simulink model "Ejercicio8_30_03_17cont"  (R2013a)
settings: Solver=ode23tb  StartTime=0.0  StopTime=0.1  RelTol=1e-3
libraries: powerlib x34
settings Model: Creator=Miguel  LastModifiedBy=Miguel

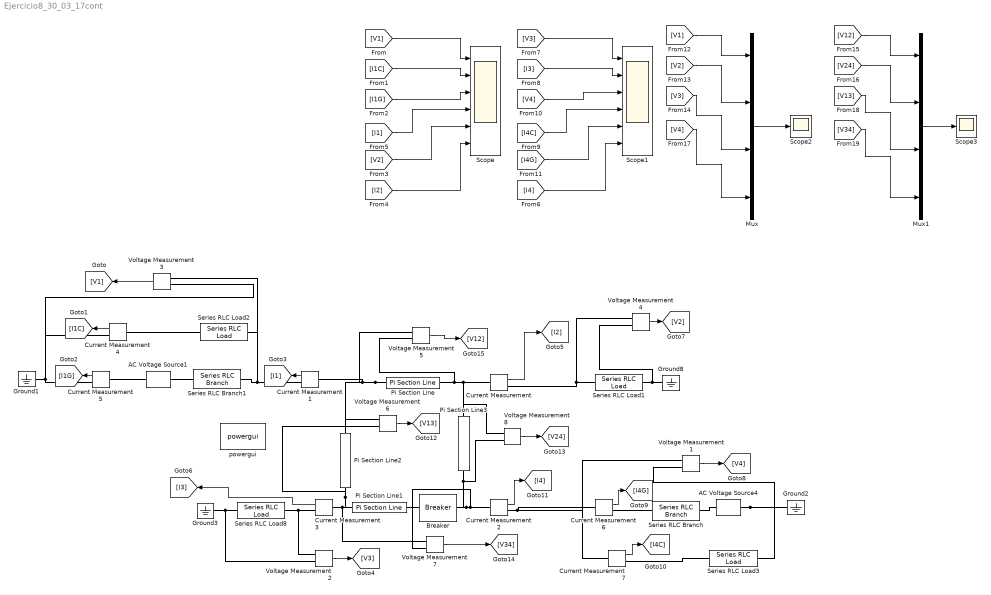
== system Ejercicio8_30_03_17cont ==
  AC Voltage Source1 : powerlib/Electrical Sources/AC Voltage Source  Amplitude=150e3*sqrt(2)  Phase=0  Frequency=60  SampleTime=0  Measurements=None
  AC Voltage Source4 : powerlib/Electrical Sources/AC Voltage Source  Amplitude=1.02*sqrt(2)*150e3  Phase=1.5231  Frequency=60  SampleTime=0  Measurements=None
  Breaker : powerlib/Elements/Breaker  BreakerResistance=0.01  InitialState=1  SnubberResistance=1e6  SnubberCapacitance=inf  SwitchingTimes=[ 1/60 ]  External=off  Measurements=None  MoreParameters=off  NoBreakLoop=off
  Current Measurement{,1..7} (8 alike) : powerlib/Measurements/Current Measurement  PhasorSimulation=off  OutputType=Complex  PSBequivalent=0
  Ground{1..3,8} (4 alike) : powerlib/Elements/Ground  LConnTagsString=a
  Mux : Mux
  Mux1 : Mux
  Pi Section Line : powerlib/Elements/Pi Section Line  LConnTagsString=__new0  RConnTagsString=__new0  Frequency=60  Resistance=0.01008*225  Inductance=0.05040/(2*pi*60)*225  Capacitance=0.05125/(pi*60*225)  Length=1  PiSections=10  Measurements=None
      settings: AttributesFormatString=\n
  Pi Section Line1 : powerlib/Elements/Pi Section Line  LConnTagsString=__new0  RConnTagsString=__new0  Frequency=60  Resistance=0.01272*225  Inductance=0.06360/(2*pi*60)*225  Capacitance=0.06375/(pi*60*225)  Length=1  PiSections=10  Measurements=All voltages and currents
      settings: AttributesFormatString=\n
  Pi Section Line2 : powerlib/Elements/Pi Section Line  LConnTagsString=__new0  RConnTagsString=__new0  Frequency=60  Resistance=0.00744*225  Inductance=0.03720/(2*pi*60)*225  Capacitance=0.03875/(pi*60*225)  Length=1  PiSections=10  Measurements=All voltages and currents
      settings: AttributesFormatString=\n
  Pi Section Line3 : powerlib/Elements/Pi Section Line  LConnTagsString=__new0  RConnTagsString=__new0  Frequency=60  Resistance=0.00744*225  Inductance=0.03720/(2*pi*60)*225  Capacitance=0.03875/(pi*60*225)  Length=1  PiSections=10  Measurements=None
      settings: AttributesFormatString=\n
  Scope : Scope  NumInputPorts=6
      settings: ShowLegends=on  YMin=-5~-5~-5~-5~-5~-5  YMax=5~5~5~5~5~5
  Scope1 : Scope  NumInputPorts=6
      settings: ShowLegends=on  YMin=-5~-5~-5~-5~-5~-5  YMax=5~5~5~5~5~5
  Scope2 : Scope
      settings: ShowLegends=on  SaveName=ScopeData2
  Scope3 : Scope
      settings: ShowLegends=on  SaveName=ScopeData3
  Series RLC Branch : powerlib/Elements/Series RLC Branch  LConnTagsString=__new0  RConnTagsString=__new0  BranchType=R  Resistance=1e-9  Inductance=1e-3  SetiL0=off  InitialCurrent=0  Capacitance=1e-6  Setx0=off  InitialVoltage=0  Measurements=None
  Series RLC Branch1 : powerlib/Elements/Series RLC Branch  LConnTagsString=__new0  RConnTagsString=__new0  BranchType=R  Resistance=1e-9  Inductance=1e-3  SetiL0=off  InitialCurrent=0  Capacitance=1e-6  Setx0=off  InitialVoltage=0  Measurements=None
  Series RLC Load1 : powerlib/Elements/Series RLC Load  LConnTagsString=a  RConnTagsString=__new0  NominalVoltage=0.9824*150e3  NominalFrequency=60  ActivePower=170e6  InductivePower=105.35e6  CapacitivePower=0  Setx0=off  InitialVoltage=0  SetiL0=off  InitialCurrent=0  Measurements=None
  Series RLC Load2 : powerlib/Elements/Series RLC Load  LConnTagsString=a  RConnTagsString=__new0  NominalVoltage=150e3  NominalFrequency=60  ActivePower=50e6  InductivePower=30.99e6  CapacitivePower=0  Setx0=off  InitialVoltage=0  SetiL0=off  InitialCurrent=0  Measurements=None
  Series RLC Load3 : powerlib/Elements/Series RLC Load  LConnTagsString=a  RConnTagsString=__new0  NominalVoltage=1.02*150e3  NominalFrequency=60  ActivePower=80e6  InductivePower=49.59e6  CapacitivePower=0  Setx0=off  InitialVoltage=0  SetiL0=off  InitialCurrent=0  Measurements=None
  Series RLC Load8 : powerlib/Elements/Series RLC Load  LConnTagsString=a  RConnTagsString=__new0  NominalVoltage=0.9690*150e3  NominalFrequency=60  ActivePower=200e6  InductivePower=123.94e6  CapacitivePower=0  Setx0=off  InitialVoltage=0  SetiL0=off  InitialCurrent=0  Measurements=Branch current
  Voltage Measurement{1..8} (8 alike) : powerlib/Measurements/Voltage Measurement  PhasorSimulation=off  OutputType=Complex  PSBequivalent=0
  powergui : powerlib/powergui  Priority=1  SimulationMode=Continuous  SolverType=Tustin  SampleTime=50e-6  frequency=60  SPID=off  DisableSnubberDevices=off  DisableRonSwitches=off  DisableVfSwitches=off  SwTol=0  Interpol=off  DisplayEquations=off  frequencyindice=60  Pbase=100e6  ErrMax=1e-4  Iterations=50  UnitsV=kV  UnitsW=MW  FunctionMessages=off  echomessages=off  HookPort=off  EnableUseOfTLC=off  x0status=blocks  RestoreLinks=warning  ResistiveCurrentMeasurement=off  Frange=[0:2:500]  Ylog=off  Xlog=on  ShowGrid=off  save=off  variable=ZData  ZoomFFT=off  StartTime=0.0  cycles=1  DisplayStyle=1  fundamental=60  FreqAxis=off  MaxFrequency=1000  frequencyindicesteady=1  RmsSteady=2  display=off  Ts=0  methode=off
  wires:
  Voltage Measurement3/1 -> [V1]
  Current Measurement4/1 -> [I1C]
  Current Measurement5/1 -> [I1G]
  Current Measurement1/1 -> [I1]
  Voltage Measurement2/1 -> [V3]
  Current Measurement3/1 -> [I3]
  Current Measurement/1 -> [I2]
  Voltage Measurement4/1 -> [V2]
  Current Measurement7/1 -> [I4C]
  Current Measurement6/1 -> [I4G]
  Voltage Measurement1/1 -> [V4]
  [V1] -> Scope/1
  [I1C] -> Scope/2
  [I1G] -> Scope/3
  [V3] -> Scope1/1
  [I3] -> Scope1/2
  [I4G] -> Scope1/5
  [I2] -> Scope/6
  [V2] -> Scope/5
  [I1] -> Scope/4
  [V4] -> Scope1/3
  [I4C] -> Scope1/4
  [I4] -> Scope1/6
  Current Measurement2/1 -> [I4]
  [V1] -> Mux/1
  [V2] -> Mux/2
  [V3] -> Mux/3
  [V4] -> Mux/4
  Mux/1 -> Scope2/1
  Voltage Measurement6/1 -> [V13]
  Voltage Measurement8/1 -> [V24]
  Voltage Measurement7/1 -> [V34]
  Voltage Measurement5/1 -> [V12]
  [V12] -> Mux1/1
  [V24] -> Mux1/2
  [V13] -> Mux1/3
  [V34] -> Mux1/4
  Mux1/1 -> Scope3/1
  connections:
  Current Measurement5/RConn1 -- Current Measurement4/RConn1 -- Voltage Measurement3/LConn2 -- Ground1/LConn1
  Current Measurement3/LConn1 -- Voltage Measurement7/LConn1 -- Voltage Measurement6/LConn2 -- Pi Section Line2/RConn1 -- Pi Section Line1/LConn1
  Current Measurement/RConn1 -- Voltage Measurement4/LConn1 -- Series RLC Load1/LConn1
  Pi Section Line3/RConn1 -- Voltage Measurement8/LConn2 -- Breaker/RConn1 -- Voltage Measurement7/LConn2 -- Current Measurement2/LConn1
  AC Voltage Source4/LConn1 -- Voltage Measurement1/LConn2 -- Ground2/LConn1 -- Series RLC Load3/RConn1
  Series RLC Load8/RConn1 -- Voltage Measurement2/LConn2 -- Ground3/LConn1
  Ground8/LConn1 -- Voltage Measurement4/LConn2 -- Series RLC Load1/RConn1
  Current Measurement1/RConn1 -- Voltage Measurement3/LConn1 -- Series RLC Load2/LConn1 -- Series RLC Branch1/RConn1
  Voltage Measurement8/LConn1 -- Pi Section Line3/LConn1 -- Current Measurement/LConn1 -- Voltage Measurement5/LConn2 -- Pi Section Line/RConn1
  Pi Section Line/LConn1 -- Voltage Measurement6/LConn1 -- Pi Section Line2/LConn1 -- Voltage Measurement5/LConn1 -- Current Measurement1/LConn1
  Current Measurement3/RConn1 -- Voltage Measurement2/LConn1 -- Series RLC Load8/LConn1
  Current Measurement2/RConn1 -- Voltage Measurement1/LConn1 -- Current Measurement6/LConn1 -- Current Measurement7/LConn1
  Current Measurement5/LConn1 -- AC Voltage Source1/LConn1
  Series RLC Branch/RConn1 -- AC Voltage Source4/RConn1
  Current Measurement4/LConn1 -- Series RLC Load2/RConn1
  Series RLC Branch/LConn1 -- Current Measurement6/RConn1
  Series RLC Load3/LConn1 -- Current Measurement7/RConn1
  Series RLC Branch1/LConn1 -- AC Voltage Source1/RConn1
  Breaker/LConn1 -- Pi Section Line1/RConn1
